simulink model "arthematic_model_M_Script"  (R2024b)
settings: Solver=VariableStepAuto  StartTime=0.0  StopTime=10.0  RelTol=1e-3
values from neighbouring files (symbols this model uses):
  A = 3    [project_1.m]
  F = 2    [project_1.m]    (also in project_m1.m = 1; project_mass_m.m = 1)
  Ti = 0.5    [project_1.m]
settings Model: Creator=vishwanth  LastModifiedBy=vishwanth

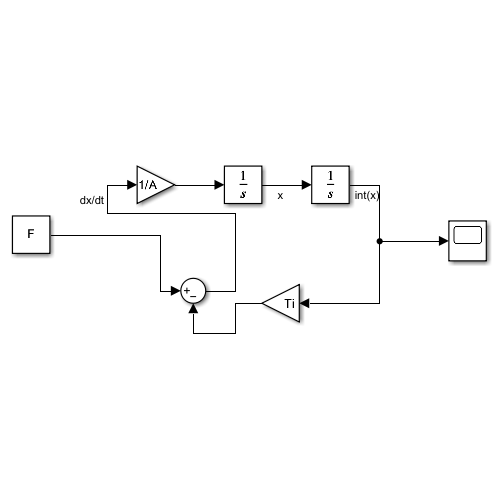
[thumbnail: Simulink's stored preview of the top-level diagram]
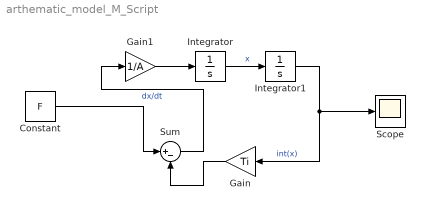
== system arthematic_model_M_Script ==
  Constant : Constant  Value=F
  Gain : Gain  Gain=Ti
  Gain1 : Gain  Gain=1/A
  Integrator : Integrator
  Integrator1 : Integrator
  Scope : Scope
  Sum : Sum  Inputs=|+-
  wires:
  Sum/1 -> Gain1/1  "dx/dt"
  Integrator/1 -> Integrator1/1  "x"
  Integrator1/1 -> Scope/1, Gain/1  "int(x)"
  Constant/1 -> Sum/1
  Gain/1 -> Sum/2
  Gain1/1 -> Integrator/1
